simulink model "L3P1"  (R2020b)
settings: Solver=VariableStepAuto  StartTime=0.0  StopTime=10.0  RelTol=1e-3
libraries: simulink x1
settings Model: Creator=jakea  LastModifiedBy=jakea

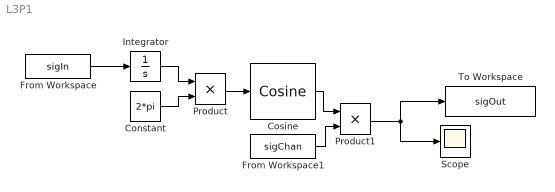
== system L3P1 ==
  Constant : Constant  Value=2*pi
  Cosine : simulink/Lookup Tables/Cosine  Formula=cos(2*pi*u)  NumDataPoints=(2^5)+1  OutputWordLength=16  InternalRulePriority=Speed
      settings: SourceProductBaseCode=SL
  From Workspace : FromWorkspace  VariableName=sigIn
  From Workspace1 : FromWorkspace  VariableName=sigChan
  Integrator : Integrator
  Product : Product
  Product1 : Product
  Scope : Scope
  To Workspace : ToWorkspace  VariableName=sigOut  SaveFormat=Timeseries  SampleTime=-1
  wires:
  From Workspace/1 -> Integrator/1
  Integrator/1 -> Product/1
  Constant/1 -> Product/2
  Product/1 -> Cosine/1
  Cosine/1 -> Product1/1
  From Workspace1/1 -> Product1/2
  Product1/1 -> To Workspace/1, Scope/1
